simulink model "example_of_virtual_subsystem"  (R2021a)
settings: Solver=FixedStepAuto  StartTime=0.0  StopTime=10.0  RelTol=1e-3
settings Model: Creator=YasserNet  LastModifiedBy=YasserNet

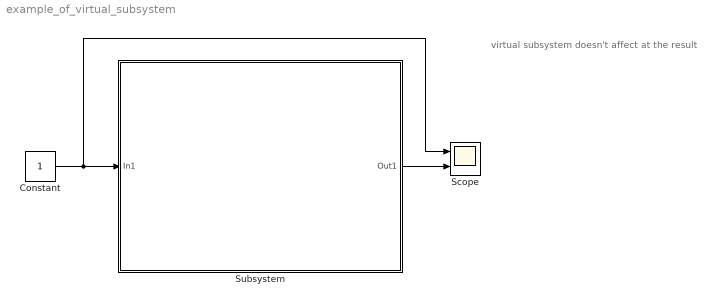
== system example_of_virtual_subsystem ==
  note: virtual subsystem doesn't affect at the result
  Constant : Constant
  Scope : Scope  NumInputPorts=2
  Subsystem : Subsystem
  wires:
  Subsystem/1(Out1) -> Scope/2
  Constant/1 -> Scope/1, Subsystem/1(In1)

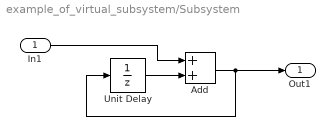
== system example_of_virtual_subsystem/Subsystem ==
  In1 : Inport
  Add : Sum
  Unit Delay : UnitDelay  SampleTime=3  HasFrameUpgradeWarning=on
  Out1 : Outport
  wires:
  Add/1 -> Out1/1, Unit Delay/1
  In1/1 -> Add/1
  Unit Delay/1 -> Add/2
